simulink model "BBB_calibration"  (R2024a)
settings: Solver=FixedStepAuto  StartTime=0.0  StopTime=30  RelTol=1e-3  EnableMultiTasking=on
libraries: bbblueSensorLib x2
settings Model: SimulationMode=external  ExtModeTrigDuration=100  Creator=Dario  LastModifiedBy=Dario
settings SolverCC: PositivePriorityOrder=on
settings DataIOCC: SaveFormat=StructureWithTime  InspectSignalLogs=on  OutputSaveName=baro
settings OptimizationCC: EnhancedBackFolding=on  PassReuseOutputArgsAs=Individual arguments  ZeroExternalMemoryAtStartup=off  ZeroInternalMemoryAtStartup=off  MaxStackSize=64  OptimizeBlockOrder=speed  DifferentSizesBufferReuse=on  OptimizationCustomize=off  EfficientTunableParamExpr=on
settings DebuggingCC: ParameterTunabilityLossMsg=error
settings HardwareCC: ProdBitPerPointer=32  ProdBitPerSizeT=32  ProdBitPerPtrDiffT=32  ProdLargestAtomicInteger=Long  ProdLargestAtomicFloat=Double  ProdWordSize=32  ProdHWDeviceType=ARM Compatible->ARM Cortex
settings SFSimCC: MATLABDynamicMemAlloc=off
settings RTWCC: Description=Embedded Coder  SystemTargetFile=ert.tlc  HardwareBoard=BeagleBone Blue  TLCOptions="-aInlineSetEventsForThisBaseRateFcn=TLC_FALSE -aSuppressMultiTaskScheduler=TLC_FALSE  -aRateBasedStepFcn=0"  TemplateMakefile=ert_default_tmf  Toolchain=GNU GCC BeagleBone Blue
settings CodeAppCC: ForceParamTrailComments=on  IgnoreCustomStorageClasses=off  OperatorAnnotations=on  SimulinkDataObjDesc=on  SFDataObjDesc=on  InsertBlockDesc=on
settings ERTTargetCC: MatFileLogging=on  SupportVariableSizeSignals=on  ExtMode=on  ExtModeMexArgs='192.168.6.2' 0 17725

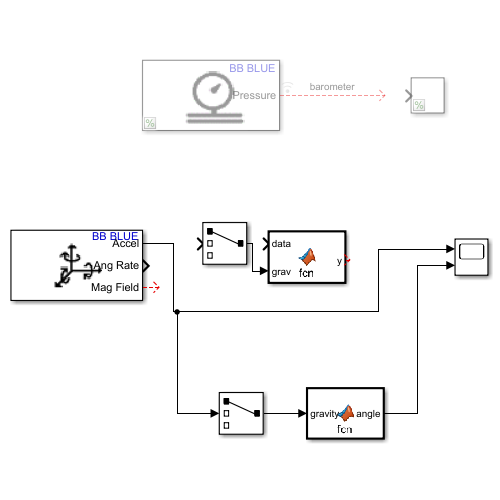
[thumbnail: Simulink's stored preview of the top-level diagram]
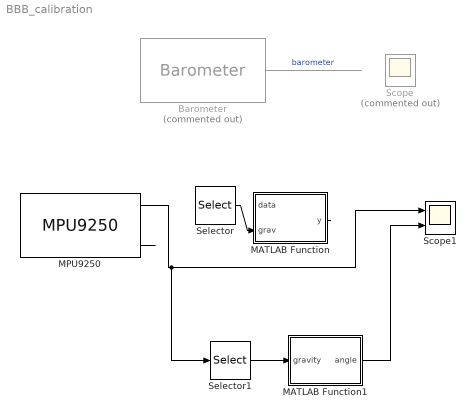
== system BBB_calibration ==
  Barometer : bbblueSensorLib/Barometer  Commented=on  OSRSelection=1  IIRFilterCoeff=Off  SampleTime=0.1
  MATLAB Function : MATLAB Function  TreatAsAtomicUnit=on
  MATLAB Function1 : MATLAB Function  TreatAsAtomicUnit=on
  MPU9250 : bbblueSensorLib/MPU9250  OperationMode=DMP  Accel=on  AngularRate=on  Ak8963Field=on  EulerAngles=off  Quat=off  AccelRange=2G  Acceldlpf=1  GyroRange=250 dps  Gyrodlpf=1  DmpOdr=200 Hz  SampleTime=0.1
  Scope : Scope  Commented=on
  Scope1 : Scope  NumInputPorts=2
  Selector : Selector  InputPortWidth=3  IndexOptions=Index vector (dialog)  Indices=[1]  OutputSizes=1
  Selector1 : Selector  InputPortWidth=3  IndexOptions=Index vector (dialog)  Indices=[1]  OutputSizes=1
  wires:
  Barometer/1 -> ?  "barometer"
  MPU9250/3 -> ?
  MPU9250/1 -> Selector1/1, Scope1/1
  MATLAB Function/1(y) -> ?
  Selector/1 -> MATLAB Function/2(grav)
  MATLAB Function1/1(angle) -> Scope1/2
  Selector1/1 -> MATLAB Function1/1(gravity)

== matlab function BBB_calibration/MATLAB Function ==
  data: data input; grav input; y output
function y = fcn(data, grav)

y = 9.174*grav;

== matlab function BBB_calibration/MATLAB Function1 ==
  data: gravity input; angle output
function angle = fcn(gravity)

angle = asin(gravity)*180/pi;
